simulink model "sampleModel653"  (R2023a)
settings: Solver=VariableStepAuto  StartTime=0.0  StopTime=10.0  RelTol=1e-3
undefined symbols (not defined in the file): DiscIntNeverNeededParam, magnitude, Newton, Raphson
libraries: simulink x238, slpidlib x68
(part 1 of 11)
settings Model: Creator=TSMC  LastModifiedBy=TSMC

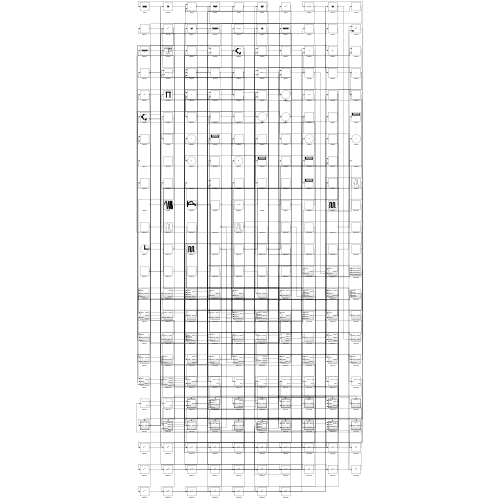
[thumbnail: Simulink's stored preview of the top-level diagram]
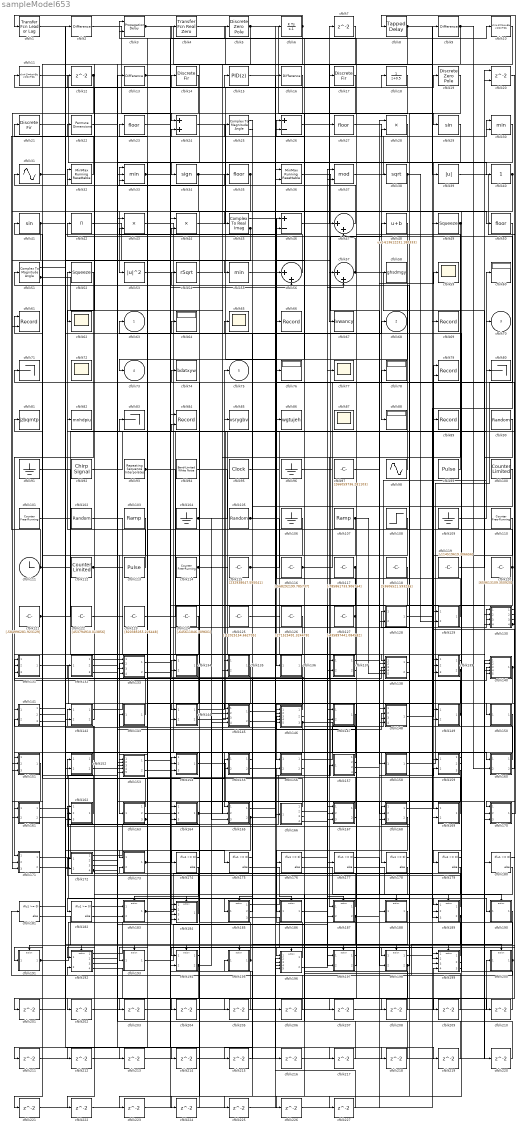
== system sampleModel653 ==
  cfblk1 : simulink/Discrete/Transfer Fcn Lead or Lag  PoleZ=0.95  ZeroZ=0.75  ICPrevOutput=0.0  ICPrevInput=0.0  DoSatur=off
  cfblk10 : DiscreteStateSpace
  cfblk100 : simulink/Sources/Counter Limited  uplimit=[350.000000]  tsamp=-1
  cfblk101 : simulink/Sources/Counter Free-Running  NumBits=[6.000000]  tsamp=-1
  cfblk102 : RandomNumber  Mean=[-2510.054914]  Variance=[85353.178897]  Seed=[22807795.000000]  SampleTime=0.1
  cfblk103 : simulink/Sources/Ramp  slope=[-6750.741057]  start=[19.762170]  InitialOutput=[686609.010483]
  cfblk{91,96,104,106,109} (5 alike) : Ground
  cfblk105 : RandomNumber  Mean=[90146.869558]  Variance=[81141.982069]  Seed=[567805556.000000]  SampleTime=0.1
  cfblk107 : simulink/Sources/Ramp  slope=[382.621128]  start=[12.088717]  InitialOutput=[440961.577354]
  cfblk108 : Step  Time=[7.000000]  Before=[-368987088.994321]  After=[512056900.809752]  SampleTime=0
  cfblk11 : DiscreteStateSpace
  cfblk110 : simulink/Sources/Counter Free-Running  NumBits=[23.000000]  tsamp=-1
  cfblk111 : Clock
  cfblk112 : simulink/Sources/Counter Limited  uplimit=[312.000000]  tsamp=-1
  cfblk113 : DiscretePulseGenerator  PulseType=Time based  Amplitude=[570954732.340234]  Period=[80381016.337612]  PulseWidth=5  PhaseDelay=[1.000000]
  cfblk114 : simulink/Sources/Counter Free-Running  NumBits=[6.000000]  tsamp=-1
  cfblk115 : Constant  Value=[232938647.595041]  SampleTime=1
  cfblk116 : Constant  Value=[-568292199.785737]  SampleTime=1
  cfblk117 : Constant  Value=[-785861733.906764]  SampleTime=1
  cfblk118 : Constant  Value=[53606521.593236]  SampleTime=1
  cfblk119 : Constant  Value=[-114519619.306656]  SampleTime=1
  cfblk{7,12,201..227} (29 alike) : Delay  SampleTime=1
  cfblk120 : Constant  Value=[659613109.350920]  SampleTime=1
  cfblk121 : Constant  Value=[-584996281.923129]  SampleTime=1
  cfblk122 : Constant  Value=[453794910.013856]  SampleTime=1
  cfblk123 : Constant  Value=[820385055.226448]  SampleTime=1
  cfblk124 : Constant  Value=[-645611846.309601]  SampleTime=1
  cfblk125 : Constant  Value=[-12025154.662705]  SampleTime=1
  cfblk126 : Constant  Value=[271525491.324478]  SampleTime=1
  cfblk127 : Constant  Value=[-435897441.084582]  SampleTime=1
  cfblk128 : Subsystem
  cfblk129 : Subsystem
  cfblk{2,9,13,16} (4 alike) : simulink/Discrete/Difference  ICPrevInput=0.0  OutMin=[]  OutMax=[]  OutDataTypeStr=Inherit: Inherit via back propagation  OutDataType=fixdt(1, 16)  OutScaling=2^-10  DoSatur=off
  cfblk130 : Subsystem
  cfblk131 : Subsystem
  cfblk132 : Subsystem
  cfblk133 : Subsystem
  cfblk134 : Subsystem
  cfblk135 : Subsystem
  cfblk136 : Subsystem
  cfblk137 : Subsystem
  cfblk138 : Subsystem
  cfblk139 : Subsystem
  cfblk14 : DiscreteFir  SampleTime=1
  cfblk140 : Subsystem
  cfblk141 : Subsystem
  cfblk142 : Subsystem
  cfblk143 : Subsystem
  cfblk144 : Subsystem
  cfblk145 : Subsystem
  cfblk146 : Subsystem
  cfblk147 : Subsystem
  cfblk148 : Subsystem
  cfblk149 : Subsystem
  cfblk15 : slpidlib/PID Controller  Controller=PID  Form=Parallel  TimeDomain=Discrete-time  UseExternalTs=off  SampleTime=1  IntegratorMethod=Forward Euler  FilterMethod=Forward Euler  ControllerParametersSource=internal  P=1  I=1  UseKiTs=off  D=0  N=100  UseFilter=on  TunerSelectOption=Transfer Function Based (PID Tuner App)  InitialConditionSource=internal  InitialConditionForIntegrator=0  InitialConditionForFilter=0  DifferentiatorICPrevScaledInput=0  ExternalReset=none  TrackingMode=off  Kt=1  LimitOutput=off  SatLimitsSource=internal  UpperSaturationLimit=inf  LowerSaturationLimit=-inf  LinearizeAsGain=off  AntiWindupMode=none  Kb=1  LimitIntegrator=off  UpperIntegratorSaturationLimit=inf  LowerIntegratorSaturationLimit=-inf  POutMin=[]  POutMax=[]  IOutMin=[]  IOutMax=[]  DOutMin=[]  DOutMax=[]  NOutMin=[]  NOutMax=[]  SumOutMin=[]  SumOutMax=[]  SaturationOutMin=[]  SaturationOutMax=[]  PParamMin=[]  PParamMax=[]  IParamMin=[]  IParamMax=[]  DParamMin=[]  DParamMax=[]  NParamMin=[]  NParamMax=[]  KbParamMin=[]  KbParamMax=[]  KtParamMin=[]  KtParamMax=[]  KbOutMin=[]  KbOutMax=[]  KtOutMin=[]  KtOutMax=[]  IntegratorOutMin=[]  IntegratorOutMax=[]  FilterOutMin=[]  FilterOutMax=[]  SumI1OutMin=[]  SumI1OutMax=[]  SumI2OutMin=[]  SumI2OutMax=[]  SumI3OutMin=[]  SumI3OutMax=[]  SumI4OutMin=[]  SumI4OutMax=[]  SumDOutMin=[]  SumDOutMax=[]  DifferentiatorOutMin=[]  DifferentiatorOutMax=[]  FilterDiffOutCoefMin=[]  FilterDiffOutCoefMax=[]  ReciprocalOutMin=[]  ReciprocalOutMax=[]  SumDenOutMin=[]  SumDenOutMax=[]  SumNumOutMin=[]  SumNumOutMax=[]  DivideOutMin=[]  DivideOutMax=[]  UdiffTsProdOutMin=[]  UdiffTsProdOutMax=[]  NTsProdOutMin=[]  NTsProdOutMax=[]  UintegralTsProdOutMin=[]  UintegralTsProdOutMax=[]  UngainTsProdOutMin=[]  UngainTsProdOutMax=[]  ClampingZeroOutDataTypeStr=Inherit: Inherit via back propagation  ClampingZeroOutMin=[]  ClampingZeroOutMax=[]  FilterDenConstantOutDataTypeStr=Inherit: Inherit via back propagation  FilterDenConstantOutMin=[]  FilterDenConstantOutMax=[]  PCopyOutDataTypeStr=Inherit: Inherit via back propagation  PCopyOutMin=[]  PCopyOutMax=[]  NCopyOutDataTypeStr=Inherit: Inherit via back propagation  NCopyOutMin=[]  NCopyOutMax=[]  IntegratorContinuousStateAttributes=''  IntegratorStateMustResolveToSignalObject=off  IntegratorRTWStateStorageClass=Auto  FilterContinuousStateAttributes=''  FilterStateMustResolveToSignalObject=off  FilterRTWStateStorageClass=Auto  ParallelPVariant=InternalParameters  IdealPVariant=Disabled  IVariant=InternalParameters  DVariant=InternalParameters  IntegratorVariant=Discrete  SatVariant=Disabled  AWVariant=Passthrough  PCopyVariant=Disabled  TRVariant=Disabled  FdbkBlocksVariant=Forward  IdealPFdbkVariant=Disabled  SatFdbkVariant=Disabled  DerivativeFilterVariant=ForwardEulerFilter  NVariant=InternalParameters  NCopyVariant=Disabled  FilterICVariant=InternalICsFilter  IntegratorICVariant=InternalICs  ExternalResetVariant=Disabled  TRSumVariant=Passthrough  SumFdbkVariant=Disabled  SumVariant=Sum_PID  TsampFilterVariant=InternalTs  TsampNgainVariant=Passthrough  TsampIntegralVariant=Disabled_SignalSpec  ExternalSaturationOutDataTypeStr=Inherit: Same as second input
      settings: LibrarySourceBlock=simulink/Discrete/Discrete PID Controller
  cfblk150 : Subsystem
  cfblk151 : Subsystem
  cfblk152 : Subsystem
  cfblk153 : Subsystem
  cfblk154 : Subsystem
  cfblk155 : Subsystem
  cfblk156 : Subsystem
  cfblk157 : Subsystem
  cfblk158 : Subsystem
  cfblk159 : Subsystem
  cfblk160 : Subsystem
  cfblk161 : Subsystem
  cfblk162 : Subsystem
  cfblk163 : Subsystem
  cfblk164 : Subsystem
  cfblk165 : Subsystem
  cfblk166 : Subsystem
  cfblk167 : Subsystem
  cfblk168 : Subsystem
  cfblk169 : Subsystem
  cfblk17 : DiscreteFir  SampleTime=1
  cfblk170 : Subsystem
  cfblk171 : Subsystem
  cfblk172 : Subsystem
  cfblk173 : Subsystem
  cfblk{174..182} (9 alike) : If  IfExpression=u1 >= 0  SampleTime=1
  cfblk18 : DiscreteTransferFcn  SampleTime=1
  cfblk183 : Subsystem  TreatAsAtomicUnit=on
  cfblk184 : Subsystem  TreatAsAtomicUnit=on
  cfblk185 : Subsystem  TreatAsAtomicUnit=on
  cfblk186 : Subsystem  TreatAsAtomicUnit=on
  cfblk187 : Subsystem  TreatAsAtomicUnit=on
  cfblk188 : Subsystem  TreatAsAtomicUnit=on
  cfblk189 : Subsystem  TreatAsAtomicUnit=on
  cfblk19 : DiscreteZeroPole  Poles=[0 0.5]  Gain=1
  cfblk190 : Subsystem  TreatAsAtomicUnit=on
  cfblk191 : Subsystem  TreatAsAtomicUnit=on
  cfblk192 : Subsystem  TreatAsAtomicUnit=on
  cfblk193 : Subsystem  TreatAsAtomicUnit=on
  cfblk194 : Subsystem  TreatAsAtomicUnit=on
  cfblk195 : Subsystem  TreatAsAtomicUnit=on
  cfblk196 : Subsystem  TreatAsAtomicUnit=on
  cfblk197 : Subsystem  TreatAsAtomicUnit=on
  cfblk198 : Subsystem  TreatAsAtomicUnit=on
  cfblk199 : Subsystem  TreatAsAtomicUnit=on
  cfblk20 : Delay  ShowEnablePort=on  SampleTime=1
      settings: InputPortMap=u0,e6
  cfblk200 : Subsystem  TreatAsAtomicUnit=on
  cfblk21 : DiscreteFir  SampleTime=1
  cfblk22 : PermuteDimensions
  cfblk{23,27,35,50} (4 alike) : Rounding
  cfblk24 : Sum
  cfblk25 : ComplexToMagnitudeAngle
  cfblk26 : Sum  Inputs=+-
  cfblk28 : Product
  cfblk29 : Trigonometry
  cfblk3 : PropagationDelay  SampleTime=1
  cfblk30 : MinMax  Inputs=2
  cfblk31 : Sin  TimeSource=Use external signal  SampleTime=0
  cfblk32 : simulink/Math Operations/MinMax Running Resettable  Function=min  vinit=0.0
  cfblk33 : MinMax  Inputs=3
  cfblk34 : Signum
  cfblk36 : simulink/Math Operations/MinMax Running Resettable  Function=min  vinit=0.0
  cfblk37 : Math  Operator=mod
  cfblk38 : Sqrt
  cfblk39 : Abs  SaturateOnIntegerOverflow=off
  cfblk4 : simulink/Discrete/Transfer Fcn Real Zero  ZeroZ=0.75  ICPrevInput=0.0  DoSatur=off
  cfblk40 : simulink/Math Operations/Slider Gain  gain=1  low=0  high=2
  cfblk41 : Trigonometry
  cfblk42 : Product  Inputs=*
  cfblk43 : Product  Inputs=**
  cfblk44 : Product  Inputs=**
  cfblk45 : ComplexToRealImag
  cfblk46 : Sum  Inputs=+-
  cfblk47 : Sum  Inputs=|++
  cfblk48 : Bias  Bias=[-613612231.180333]  SaturateOnIntegerOverflow=off
  cfblk49 : Squeeze
  cfblk5 : DiscreteZeroPole  Poles=[0 0.5]  Gain=1
  cfblk51 : ComplexToMagnitudeAngle
  cfblk52 : Squeeze
  cfblk53 : Math  Operator=magnitude^2
  cfblk54 : Sqrt  Operator=rSqrt  AlgorithmType=Newton-Raphson
  cfblk55 : MinMax
  cfblk56 : Sum  Inputs=|++
  cfblk57 : Sum  Inputs=|++
  cfblk58 : ToWorkspace  VariableName=ghsdmgy  SaveFormat=Timeseries  SampleTime=-1
  cfblk{59,62,65,72,77,87} (6 alike) : Scope
      cfblk72 settings: Floating=on
      cfblk87 settings: Floating=on
  cfblk6 : DiscreteIntegrator  ICPrevOutput=DiscIntNeverNeededParam  ICPrevScaledInput=DiscIntNeverNeededParam
  cfblk{60,64,76,78,88} (5 alike) : Display
  cfblk61 : Record  FileSettingsInternal="{\"entries\":[{\"content\":{\"excelSettings\":{\"content\":{},\"type\":\"Streamout.ExcelSettings\"}},\"type\":\"Streamout.FileSettingStorage\",\"uuid\":\"\"}],\"packageUris\":[\"http:\\/\\/schema.mathworks.com\\/mf0\\/streamout_blocks\\/R2020a\"],\"version\":\"1.0\"}"  Layout=[1 1]  SignalsInternal="{\"entries\":[{\"content\":{\"signals\":[{\"content\":{\"blockPath\":[],\"dimensions\":[1],\"domain\":\"\",\"lineColor\":\"#a2142f\",\"plots\":[1],\"port\":1,\"signalID\":35743,\"signalName\":\"XY Graph:1\"},\"type\":\"RecordBlkView.Signal\",\"uuid\":\"\"},{\"content\":{\"blockPath\":[],\"dimensions\":[1],\"domain\":\"\",\"lineColor\":\"#139fff\",\"plots\":[1],\"port\":2,\"signalID\":35746,\"signalName\":\"XY Graph:2\"},\"type\":\"RecordBlkView.Signal\",\"uuid\":\"\"}]},\"type\":\"RecordBlkView.InputSignals\",\"uuid\":\"\"}],\"packageUris\":[\"http:\\/\\/schema.mathworks.com\\/mf0\\/streamout_blocks\\/R2020a\"],\"version\":\"1.0\"}"  VisualizationBindings="{\"xyplotplugin\":{\"info\":[{\"series\":[{\"bindingParametersList\":[{\"parameter\":\"X-Axis\",\"signalID\":35743,\"signalName\":\"XY Graph:1\"},{\"parameter\":\"Y-Axis\",\"signalID\":35746,\"signalName\":\"XY Graph:2\"}],\"seriesID\":38443}],\"subplotID\":1}]}}"  CompatibilityTag=XY
  cfblk66 : Record  FileSettingsInternal="{\"entries\":[{\"content\":{\"excelSettings\":{\"content\":{},\"type\":\"Streamout.ExcelSettings\"}},\"type\":\"Streamout.FileSettingStorage\",\"uuid\":\"\"}],\"packageUris\":[\"http:\\/\\/schema.mathworks.com\\/mf0\\/streamout_blocks\\/R2020a\"],\"version\":\"1.0\"}"  SignalsInternal="{\"entries\":[{\"content\":{},\"type\":\"RecordBlkView.InputSignals\",\"uuid\":\"\"}],\"packageUris\":[\"http:\\/\\/schema.mathworks.com\\/mf0\\/streamout_blocks\\/R2020a\"],\"version\":\"1.0\"}"  VisualizationBindings="{\"sparklinesplugin\":{\"info\":[{\"bindingParametersList\":[],\"subplotID\":1}]}}"
  cfblk67 : ToWorkspace  VariableName=lvwancy  SaveFormat=Timeseries  SampleTime=-1
  cfblk69 : Record  FileSettingsInternal="{\"entries\":[{\"content\":{\"excelSettings\":{\"content\":{},\"type\":\"Streamout.ExcelSettings\"}},\"type\":\"Streamout.FileSettingStorage\",\"uuid\":\"\"}],\"packageUris\":[\"http:\\/\\/schema.mathworks.com\\/mf0\\/streamout_blocks\\/R2020a\"],\"version\":\"1.0\"}"  SignalsInternal="{\"entries\":[{\"content\":{},\"type\":\"RecordBlkView.InputSignals\",\"uuid\":\"\"}],\"packageUris\":[\"http:\\/\\/schema.mathworks.com\\/mf0\\/streamout_blocks\\/R2020a\"],\"version\":\"1.0\"}"  VisualizationBindings="{\"sparklinesplugin\":{\"info\":[{\"bindingParametersList\":[],\"subplotID\":1}]}}"
  cfblk71 : Terminator
  cfblk74 : ToWorkspace  VariableName=bdatxyw  SaveFormat=Timeseries  SampleTime=-1
  cfblk79 : Record  FileSettingsInternal="{\"entries\":[{\"content\":{\"excelSettings\":{\"content\":{},\"type\":\"Streamout.ExcelSettings\"}},\"type\":\"Streamout.FileSettingStorage\",\"uuid\":\"\"}],\"packageUris\":[\"http:\\/\\/schema.mathworks.com\\/mf0\\/streamout_blocks\\/R2020a\"],\"version\":\"1.0\"}"  Layout=[1 1]  SignalsInternal="{\"entries\":[{\"content\":{\"signals\":[{\"content\":{\"blockPath\":[],\"dimensions\":[1],\"domain\":\"\",\"lineColor\":\"#a2142f\",\"plots\":[1],\"port\":1,\"signalID\":35751,\"signalName\":\"XY Graph:1\"},\"type\":\"RecordBlkView.Signal\",\"uuid\":\"\"},{\"content\":{\"blockPath\":[],\"dimensions\":[1],\"domain\":\"\",\"lineColor\":\"#139fff\",\"plots\":[1],\"port\":2,\"signalID\":35754,\"signalName\":\"XY Graph:2\"},\"type\":\"RecordBlkView.Signal\",\"uuid\":\"\"}]},\"type\":\"RecordBlkView.InputSignals\",\"uuid\":\"\"}],\"packageUris\":[\"http:\\/\\/schema.mathworks.com\\/mf0\\/streamout_blocks\\/R2020a\"],\"version\":\"1.0\"}"  VisualizationBindings="{\"xyplotplugin\":{\"info\":[{\"series\":[{\"bindingParametersList\":[{\"parameter\":\"X-Axis\",\"signalID\":35751,\"signalName\":\"XY Graph:1\"},{\"parameter\":\"Y-Axis\",\"signalID\":35754,\"signalName\":\"XY Graph:2\"}],\"seriesID\":62220}],\"subplotID\":1}]}}"  CompatibilityTag=XY
  cfblk8 : simulink/Discrete/Tapped Delay  vinit=0.0  samptime=-1  NumDelays=1  DelayOrder=Oldest  includeCurrent=off
  cfblk80 : Terminator
  cfblk81 : ToWorkspace  VariableName=jzbqmtp  SaveFormat=Timeseries  SampleTime=-1
  cfblk82 : ToWorkspace  VariableName=mnhdpiu  SaveFormat=Timeseries  SampleTime=-1
  cfblk83 : Terminator
  cfblk84 : Record  FileSettingsInternal="{\"entries\":[{\"content\":{\"excelSettings\":{\"content\":{},\"type\":\"Streamout.ExcelSettings\"}},\"type\":\"Streamout.FileSettingStorage\",\"uuid\":\"\"}],\"packageUris\":[\"http:\\/\\/schema.mathworks.com\\/mf0\\/streamout_blocks\\/R2020a\"],\"version\":\"1.0\"}"  Layout=[1 1]  SignalsInternal="{\"entries\":[{\"content\":{\"signals\":[{\"content\":{\"blockPath\":[],\"dimensions\":[1],\"domain\":\"\",\"lineColor\":\"#a2142f\",\"plots\":[1],\"port\":1,\"signalID\":35759,\"signalName\":\"XY Graph:1\"},\"type\":\"RecordBlkView.Signal\",\"uuid\":\"\"},{\"content\":{\"blockPath\":[],\"dimensions\":[1],\"domain\":\"\",\"lineColor\":\"#139fff\",\"plots\":[1],\"port\":2,\"signalID\":35762,\"signalName\":\"XY Graph:2\"},\"type\":\"RecordBlkView.Signal\",\"uuid\":\"\"}]},\"type\":\"RecordBlkView.InputSignals\",\"uuid\":\"\"}],\"packageUris\":[\"http:\\/\\/schema.mathworks.com\\/mf0\\/streamout_blocks\\/R2020a\"],\"version\":\"1.0\"}"  VisualizationBindings="{\"xyplotplugin\":{\"info\":[{\"series\":[{\"bindingParametersList\":[{\"parameter\":\"X-Axis\",\"signalID\":35759,\"signalName\":\"XY Graph:1\"},{\"parameter\":\"Y-Axis\",\"signalID\":35762,\"signalName\":\"XY Graph:2\"}],\"seriesID\":44318}],\"subplotID\":1}]}}"  CompatibilityTag=XY
  cfblk85 : ToWorkspace  VariableName=vsrygbv  SaveFormat=Timeseries  SampleTime=-1
  cfblk86 : ToWorkspace  VariableName=wgtujeh  SaveFormat=Timeseries  SampleTime=-1
  cfblk89 : Record  FileSettingsInternal="{\"entries\":[{\"content\":{\"excelSettings\":{\"content\":{},\"type\":\"Streamout.ExcelSettings\"}},\"type\":\"Streamout.FileSettingStorage\",\"uuid\":\"\"}],\"packageUris\":[\"http:\\/\\/schema.mathworks.com\\/mf0\\/streamout_blocks\\/R2020a\"],\"version\":\"1.0\"}"  SignalsInternal="{\"entries\":[{\"content\":{},\"type\":\"RecordBlkView.InputSignals\",\"uuid\":\"\"}],\"packageUris\":[\"http:\\/\\/schema.mathworks.com\\/mf0\\/streamout_blocks\\/R2020a\"],\"version\":\"1.0\"}"  VisualizationBindings="{\"sparklinesplugin\":{\"info\":[{\"bindingParametersList\":[],\"subplotID\":1}]}}"
  cfblk90 : RandomNumber  Mean=[81983.003222]  Variance=[14220.056045]  Seed=[398225088.000000]  SampleTime=0.1
  cfblk92 : simulink/Sources/Chirp Signal  f1=[-164452371.357946]  T=[-247135005.835432]  f2=[-278737308.417213]
  cfblk93 : simulink/Sources/Repeating Sequence Interpolated  OutValues=[-576342041.016997, 372535724.917428, 895075316.780555, 485237690.974424, -398965901.988009]  TimeValues=[0 0.1 0.5 0.6 1].'  LookUpMeth=Use Input Above  tsamp=0.01  OutMin=[]  OutMax=[]  OutDataTypeStr=double  OutputDataTypeScalingMode=double  OutDataType=fixdt(0,8)  OutScaling=2^-10
  cfblk94 : simulink/Sources/Band-Limited White Noise  Cov=[3370681036.098789]  Ts=0.1  seed=[9057757928.000000]
  cfblk95 : DigitalClock
  cfblk97 : Constant  Value=[266059736.281103]  SampleTime=1
  cfblk98 : Sin  Amplitude=[-992289981.566664]  Bias=[-48582616.764596]  SampleTime=0
  cfblk99 : DiscretePulseGenerator  PulseType=Time based  Amplitude=[883932493.982102]  Period=[82177714.004234]  PulseWidth=5  PhaseDelay=[9.000000]
  cfblk63 : Outport
  cfblk68 : Outport  Port=2
  cfblk70 : Outport  Port=3
  cfblk73 : Outport  Port=4
  cfblk75 : Outport  Port=5
  wires:
  cfblk192/1(cfblk2) -> cfblk154/1(cfblk1)
  cfblk98/1 -> cfblk51/1
  cfblk2/1 -> cfblk24/1
  cfblk156/1(cfblk2) -> cfblk60/1
  cfblk44/1 -> cfblk19/1
  cfblk136/1(cfblk2) -> cfblk156/1(cfblk1)
  cfblk111/1 -> cfblk24/2, cfblk153/5(cfblk15)
  cfblk158/1(cfblk2) -> cfblk42/1
  cfblk45/1 -> cfblk136/1(cfblk1)
  cfblk127/1 -> cfblk46/1, cfblk145/1(cfblk1)
  cfblk51/1 -> cfblk2/1
  cfblk169/1(cfblk2) -> cfblk71/1
  cfblk99/1 -> cfblk32/1
  cfblk39/1 -> cfblk150/1(cfblk1)
  cfblk109/1 -> cfblk70/1
  cfblk49/1 -> cfblk187/1(cfblk1), cfblk145/3(cfblk14)
  cfblk118/1 -> cfblk154/2(cfblk12)
  cfblk147/1(cfblk2) -> cfblk174/1
  cfblk196/1(cfblk2) -> cfblk156/2(cfblk15)
  cfblk107/1 -> cfblk163/1(cfblk1), cfblk138/5(cfblk16)
  cfblk126/1 -> cfblk171/1(cfblk1)
  cfblk26/1 -> cfblk7/1
  cfblk27/1 -> cfblk88/1
  cfblk43/1 -> cfblk197/1(cfblk1)
  cfblk144/1(cfblk2) -> cfblk75/1
  cfblk129/1(cfblk2) -> cfblk26/1
  cfblk23/1 -> cfblk164/1(cfblk1)
  cfblk170/1(cfblk2) -> cfblk8/1
  cfblk11/1 -> cfblk169/1(cfblk1)
  cfblk148/1(cfblk2) -> cfblk79/1
  cfblk156/2(cfblk16) -> cfblk32/2
  cfblk197/2(cfblk10) -> cfblk15/1
  cfblk172/1(cfblk2) -> cfblk48/1
  cfblk135/1(cfblk2) -> cfblk164/2(cfblk7)
  cfblk116/1 -> cfblk20/1, cfblk89/1
  cfblk150/1(cfblk2) -> cfblk165/1(cfblk1)
  cfblk53/1 -> cfblk178/1
  cfblk168/1(cfblk2) -> cfblk49/1
  cfblk119/1 -> cfblk20/2
  cfblk160/1(cfblk2) -> cfblk54/1
  cfblk41/1 -> cfblk160/1(cfblk1), cfblk171/3(cfblk9)
  cfblk139/1(cfblk2) -> cfblk154/3(cfblk13)
  cfblk47/1 -> cfblk22/1
  cfblk34/1 -> cfblk86/1, cfblk144/2(cfblk7)
  cfblk113/1 -> cfblk52/1
  cfblk91/1 -> cfblk166/1(cfblk1)
  cfblk31/1 -> cfblk14/1, cfblk148/4(cfblk8)
  cfblk162/1(cfblk2) -> cfblk61/1
  cfblk32/1 -> cfblk21/1
  cfblk7/1 -> cfblk34/1
  cfblk105/1 -> cfblk65/1, cfblk140/2(cfblk7)
  cfblk183/1(cfblk2) -> cfblk69/1, cfblk140/3(cfblk8)
  cfblk138/1(cfblk2) -> cfblk182/1
  cfblk184/1(cfblk2) -> cfblk142/1(cfblk1)
  cfblk3/1 -> cfblk39/1, cfblk196/1(cfblk1)
  cfblk51/2 -> cfblk165/2(cfblk8), cfblk46/2
  cfblk189/1(cfblk2) -> cfblk168/1(cfblk1)
  cfblk4/1 -> cfblk67/1
  cfblk30/1 -> cfblk76/1
  cfblk6/1 -> cfblk1/1, cfblk135/2(cfblk10)
  cfblk138/2(cfblk17) -> cfblk198/1(cfblk1)
  cfblk96/1 -> cfblk9/1
  cfblk106/1 -> cfblk191/1(cfblk1)
  cfblk193/1(cfblk2) -> cfblk167/1(cfblk1)
  cfblk5/1 -> cfblk29/1, cfblk33/2
  cfblk196/2(cfblk17) -> cfblk77/1
  cfblk133/1(cfblk2) -> cfblk164/3(cfblk8)
  cfblk124/1 -> cfblk193/1(cfblk1)
  cfblk190/1(cfblk2) -> cfblk181/1
  cfblk165/1(cfblk2) -> cfblk198/2(cfblk16)
  cfblk167/1(cfblk2) -> cfblk143/1(cfblk1)
  cfblk93/1 -> cfblk138/1(cfblk1), cfblk130/4(cfblk13)
  cfblk134/1(cfblk2) -> cfblk173/1(cfblk1)
  cfblk168/2(cfblk12) -> cfblk186/1(cfblk1)
  cfblk29/1 -> cfblk153/1(cfblk1)
  cfblk35/1 -> cfblk144/1(cfblk1), cfblk33/3
  cfblk38/1 -> cfblk53/1, cfblk129/2(cfblk13)
  cfblk142/1(cfblk2) -> cfblk149/1(cfblk1)
  cfblk46/1 -> cfblk17/1
  cfblk200/1(cfblk2) -> cfblk128/1(cfblk1), cfblk192/2(cfblk14)
  cfblk40/1 -> cfblk61/2, cfblk209/1
  cfblk130/3(cfblk15) -> cfblk194/1(cfblk1)
  cfblk52/1 -> cfblk141/1(cfblk1)
  cfblk92/1 -> cfblk44/1
  cfblk131/1(cfblk2) -> cfblk146/1(cfblk1)
  cfblk145/1(cfblk2) -> cfblk78/1
  cfblk139/2(cfblk16) -> cfblk64/1, cfblk207/1
  cfblk33/1 -> cfblk28/2, cfblk47/1, cfblk218/1
  cfblk185/1(cfblk2) -> cfblk190/1(cfblk1)
  cfblk140/1(cfblk2) -> cfblk179/1, cfblk213/1
  cfblk112/1 -> cfblk12/1, cfblk187/2(cfblk6)
  cfblk37/1 -> cfblk30/1
  cfblk9/1 -> cfblk151/1(cfblk1), cfblk160/2(cfblk8)
  cfblk137/1(cfblk2) -> cfblk59/1
  cfblk157/1(cfblk2) -> cfblk63/1
  cfblk146/1(cfblk2) -> cfblk82/1
  cfblk104/1 -> cfblk16/1, cfblk165/3(cfblk9)
  cfblk154/1(cfblk2) -> cfblk197/2(cfblk9)
  cfblk120/1 -> cfblk23/1, cfblk147/2(cfblk14)
  cfblk45/2 -> cfblk151/2(cfblk10), cfblk43/2
  cfblk189/2(cfblk10) -> cfblk83/1, cfblk131/3(cfblk15), cfblk227/1
  cfblk28/1 -> cfblk153/2(cfblk12)
  cfblk25/1 -> cfblk45/1
  cfblk123/1 -> cfblk36/1
  cfblk187/1(cfblk2) -> cfblk141/2(cfblk5)
  cfblk195/1(cfblk2) -> cfblk184/2(cfblk13), cfblk162/2(cfblk12)
  cfblk165/2(cfblk10) -> cfblk36/2, cfblk172/2(cfblk6)
  cfblk192/2(cfblk15) -> cfblk44/2
  cfblk173/1(cfblk2) -> cfblk85/1, cfblk33/1
  cfblk153/1(cfblk2) -> cfblk130/1(cfblk1)
  cfblk14/1 -> cfblk161/1(cfblk1)
  cfblk48/1 -> cfblk73/1
  cfblk199/1(cfblk2) -> cfblk66/1
  cfblk145/2(cfblk16) -> cfblk30/2
  cfblk17/1 -> cfblk183/2(cfblk8)
  cfblk108/1 -> cfblk146/2(cfblk9)
  cfblk117/1 -> cfblk167/2(cfblk15), cfblk194/2(cfblk12)
  cfblk171/1(cfblk2) -> cfblk84/1
  cfblk161/1(cfblk2) -> cfblk189/1(cfblk1)
  cfblk146/2(cfblk13) -> cfblk134/1(cfblk1)
  cfblk166/1(cfblk2) -> cfblk152/1(cfblk1)
  cfblk141/1(cfblk2) -> cfblk68/1
  cfblk186/1(cfblk2) -> cfblk37/1
  cfblk94/1 -> cfblk169/2(cfblk7)
  cfblk101/1 -> cfblk26/2
  cfblk12/1 -> cfblk161/2(cfblk15), cfblk151/3(cfblk11)
  cfblk149/1(cfblk2) -> cfblk133/2(cfblk7), cfblk135/1(cfblk1)
  cfblk185/2(cfblk13) -> cfblk134/2(cfblk9)
  cfblk164/1(cfblk2) -> cfblk168/2(cfblk10), cfblk140/5(cfblk10)
  cfblk36/1 -> cfblk128/2(cfblk17)
  cfblk152/1(cfblk2) -> cfblk81/1
  cfblk133/2(cfblk10) -> cfblk175/1
  cfblk171/2(cfblk10) -> cfblk43/1
  cfblk18/1 -> cfblk56/1
  cfblk191/1(cfblk2) -> cfblk5/1, cfblk18/1, cfblk146/4(cfblk11)
  cfblk97/1 -> cfblk158/1(cfblk1)
  cfblk24/1 -> cfblk50/1
  cfblk192/3(cfblk16) -> cfblk25/1
  cfblk121/1 -> cfblk37/2, cfblk80/1
  cfblk157/2(cfblk13) -> cfblk146/3(cfblk10)
  cfblk130/4(cfblk16) -> cfblk74/1, cfblk84/2
  cfblk110/1 -> cfblk189/2(cfblk8)
  cfblk55/1 -> cfblk189/3(cfblk9)
  cfblk172/2(cfblk7) -> cfblk13/1
  cfblk185/3(cfblk14) -> cfblk199/2(cfblk13)
  cfblk57/1 -> cfblk180/1, cfblk47/2
  cfblk142/2(cfblk16) -> cfblk31/1
  cfblk1/1 -> cfblk57/1
  cfblk115/1 -> cfblk57/2, cfblk58/1
  cfblk137/2(cfblk14) -> cfblk4/1
  cfblk20/1 -> cfblk170/1(cfblk1)
  cfblk103/1 -> cfblk153/4(cfblk14)
  cfblk160/2(cfblk9) -> cfblk129/1(cfblk1)
  cfblk166/2(cfblk8) -> cfblk139/1(cfblk1)
  cfblk56/1 -> cfblk3/1
  cfblk157/3(cfblk14) -> cfblk79/2
  cfblk187/2(cfblk7) -> cfblk159/2(cfblk6), cfblk226/1
  cfblk13/1 -> cfblk10/1, cfblk140/4(cfblk9)
  cfblk128/1(cfblk2) -> cfblk139/2(cfblk14)
  cfblk102/1 -> cfblk177/1
  cfblk42/1 -> cfblk55/1
  cfblk50/1 -> cfblk139/3(cfblk15)
  cfblk141/2(cfblk6) -> cfblk137/1(cfblk1)
  cfblk54/1 -> cfblk170/2(cfblk13)
  cfblk122/1 -> cfblk148/1(cfblk1)
  cfblk90/1 -> cfblk130/2(cfblk11)
  cfblk16/1 -> cfblk152/2(cfblk13)
  cfblk146/3(cfblk14) -> cfblk220/1, cfblk221/1
  cfblk152/2(cfblk14) -> cfblk35/1
  cfblk143/1(cfblk2) -> cfblk132/1(cfblk1)
  cfblk166/3(cfblk9) -> cfblk3/2
  cfblk172/3(cfblk8) -> cfblk148/2(cfblk6)
  cfblk100/1 -> cfblk185/1(cfblk1)
  cfblk198/1(cfblk2) -> cfblk159/1(cfblk1)
  cfblk125/1 -> cfblk147/1(cfblk1)
  cfblk198/2(cfblk17) -> cfblk162/1(cfblk1), cfblk225/1
  cfblk8/1 -> cfblk40/1, cfblk162/3(cfblk13)
  cfblk151/1(cfblk2) -> cfblk171/2(cfblk8)
  cfblk95/1 -> cfblk38/1
  cfblk161/2(cfblk16) -> cfblk155/1(cfblk1)
  cfblk159/2(cfblk7) -> cfblk167/3(cfblk16)
  cfblk199/2(cfblk16) -> cfblk155/2(cfblk9)
  cfblk172/4(cfblk9) -> cfblk148/3(cfblk7), cfblk192/1(cfblk1), cfblk222/1
  cfblk132/1(cfblk2) -> cfblk170/3(cfblk14)
  cfblk157/4(cfblk15) -> cfblk131/1(cfblk1)
  cfblk166/4(cfblk10) -> cfblk130/3(cfblk12)
  cfblk144/2(cfblk8) -> cfblk6/1
  cfblk10/1 -> cfblk62/1
  cfblk155/2(cfblk10) -> cfblk157/1(cfblk1)
  cfblk163/1(cfblk2) -> cfblk41/1
  cfblk194/2(cfblk13) -> cfblk145/2(cfblk13), cfblk212/1
  cfblk167/2(cfblk17) -> cfblk11/1
  cfblk199/3(cfblk17) -> cfblk172/1(cfblk1)
  cfblk163/2(cfblk8) -> cfblk56/2
  cfblk114/1 -> cfblk137/2(cfblk13), cfblk145/4(cfblk15)
  cfblk132/3(cfblk14) -> cfblk27/1
  cfblk163/3(cfblk9) -> cfblk133/4(cfblk9), cfblk131/2(cfblk14)
  cfblk141/3(cfblk7) -> cfblk138/3(cfblk14)
  cfblk174/1 -> cfblk183/Action
  cfblk174/2 -> cfblk184/Action
  cfblk175/1 -> cfblk185/Action
  cfblk175/2 -> cfblk186/Action
  cfblk176/1 -> cfblk187/Action
  cfblk176/2 -> cfblk188/Action
  cfblk177/1 -> cfblk189/Action
  cfblk177/2 -> cfblk190/Action
  cfblk178/1 -> cfblk191/Action
  cfblk178/2 -> cfblk192/Action
  cfblk179/1 -> cfblk193/Action
  cfblk179/2 -> cfblk194/Action
  cfblk180/1 -> cfblk195/Action
  cfblk180/2 -> cfblk196/Action
  cfblk181/1 -> cfblk197/Action
  cfblk181/2 -> cfblk198/Action
  cfblk182/1 -> cfblk199/Action
  cfblk182/2 -> cfblk200/Action
  cfblk155/1(cfblk2) -> cfblk201/1
  cfblk201/1 -> cfblk142/2(cfblk15)
  cfblk130/1(cfblk2) -> cfblk202/1
  cfblk202/1 -> cfblk199/1(cfblk1)
  cfblk130/2(cfblk14) -> cfblk203/1
  cfblk203/1 -> cfblk200/1(cfblk1)
  cfblk197/1(cfblk2) -> cfblk204/1
  cfblk204/1 -> cfblk188/1(cfblk1)
  cfblk188/1(cfblk2) -> cfblk205/1
  cfblk205/1 -> cfblk184/3(cfblk14)
  cfblk15/1 -> cfblk206/1
  cfblk206/1 -> cfblk153/3(cfblk13)
  cfblk207/1 -> cfblk199/4(cfblk15)
  cfblk19/1 -> cfblk208/1
  cfblk208/1 -> cfblk183/1(cfblk1)
  cfblk209/1 -> cfblk146/5(cfblk12)
  cfblk132/2(cfblk13) -> cfblk210/1
  cfblk210/1 -> cfblk173/2(cfblk7)
  cfblk194/1(cfblk2) -> cfblk211/1
  cfblk211/1 -> cfblk140/1(cfblk1)
  cfblk212/1 -> cfblk168/3(cfblk11)
  cfblk213/1 -> cfblk196/3(cfblk14)
  cfblk21/1 -> cfblk214/1
  cfblk214/1 -> cfblk28/1
  cfblk25/2 -> cfblk215/1
  cfblk215/1 -> cfblk195/1(cfblk1)
  cfblk192/4(cfblk17) -> cfblk216/1
  cfblk216/1 -> cfblk138/2(cfblk13)
  cfblk153/2(cfblk16) -> cfblk217/1
  cfblk217/1 -> cfblk176/1
  cfblk218/1 -> cfblk196/2(cfblk13)
  cfblk22/1 -> cfblk219/1
  cfblk219/1 -> cfblk133/1(cfblk1)
  cfblk220/1 -> cfblk133/3(cfblk8)
  cfblk221/1 -> cfblk138/4(cfblk15)
  cfblk222/1 -> cfblk199/3(cfblk14)
  cfblk159/1(cfblk2) -> cfblk223/1
  cfblk223/1 -> cfblk184/1(cfblk1)
  cfblk159/3(cfblk8) -> cfblk224/1
  cfblk224/1 -> cfblk184/4(cfblk15)
  cfblk225/1 -> cfblk196/5(cfblk16)
  cfblk226/1 -> cfblk149/2(cfblk15)
  cfblk227/1 -> cfblk196/4(cfblk15)

== system sampleModel653/cfblk128 ==
  cfblk1 : Inport
  cfblk17 : Inport  Port=2
  cfblk10 : Math  Operator=mod
  cfblk11 : Constant  Value=[-332037826.006319]  SampleTime=1
  cfblk12 : Subsystem
  cfblk13 : Subsystem
  cfblk14 : Subsystem
  cfblk15 : Subsystem
  cfblk16 : Subsystem
  cfblk18 : Delay  SampleTime=1
  cfblk19 : Delay  SampleTime=1
  cfblk3 : slpidlib/PID Controller  Controller=PID  Form=Parallel  TimeDomain=Discrete-time  UseExternalTs=off  SampleTime=1  IntegratorMethod=Forward Euler  FilterMethod=Forward Euler  ControllerParametersSource=internal  P=1  I=1  UseKiTs=off  D=0  N=100  UseFilter=on  TunerSelectOption=Transfer Function Based (PID Tuner App)  InitialConditionSource=internal  InitialConditionForIntegrator=0  InitialConditionForFilter=0  DifferentiatorICPrevScaledInput=0  ExternalReset=none  TrackingMode=off  Kt=1  LimitOutput=off  SatLimitsSource=internal  UpperSaturationLimit=inf  LowerSaturationLimit=-inf  LinearizeAsGain=off  AntiWindupMode=none  Kb=1  LimitIntegrator=off  UpperIntegratorSaturationLimit=inf  LowerIntegratorSaturationLimit=-inf  POutMin=[]  POutMax=[]  IOutMin=[]  IOutMax=[]  DOutMin=[]  DOutMax=[]  NOutMin=[]  NOutMax=[]  SumOutMin=[]  SumOutMax=[]  SaturationOutMin=[]  SaturationOutMax=[]  PParamMin=[]  PParamMax=[]  IParamMin=[]  IParamMax=[]  DParamMin=[]  DParamMax=[]  NParamMin=[]  NParamMax=[]  KbParamMin=[]  KbParamMax=[]  KtParamMin=[]  KtParamMax=[]  KbOutMin=[]  KbOutMax=[]  KtOutMin=[]  KtOutMax=[]  IntegratorOutMin=[]  IntegratorOutMax=[]  FilterOutMin=[]  FilterOutMax=[]  SumI1OutMin=[]  SumI1OutMax=[]  SumI2OutMin=[]  SumI2OutMax=[]  SumI3OutMin=[]  SumI3OutMax=[]  SumI4OutMin=[]  SumI4OutMax=[]  SumDOutMin=[]  SumDOutMax=[]  DifferentiatorOutMin=[]  DifferentiatorOutMax=[]  FilterDiffOutCoefMin=[]  FilterDiffOutCoefMax=[]  ReciprocalOutMin=[]  ReciprocalOutMax=[]  SumDenOutMin=[]  SumDenOutMax=[]  SumNumOutMin=[]  SumNumOutMax=[]  DivideOutMin=[]  DivideOutMax=[]  UdiffTsProdOutMin=[]  UdiffTsProdOutMax=[]  NTsProdOutMin=[]  NTsProdOutMax=[]  UintegralTsProdOutMin=[]  UintegralTsProdOutMax=[]  UngainTsProdOutMin=[]  UngainTsProdOutMax=[]  ClampingZeroOutDataTypeStr=Inherit: Inherit via back propagation  ClampingZeroOutMin=[]  ClampingZeroOutMax=[]  FilterDenConstantOutDataTypeStr=Inherit: Inherit via back propagation  FilterDenConstantOutMin=[]  FilterDenConstantOutMax=[]  PCopyOutDataTypeStr=Inherit: Inherit via back propagation  PCopyOutMin=[]  PCopyOutMax=[]  NCopyOutDataTypeStr=Inherit: Inherit via back propagation  NCopyOutMin=[]  NCopyOutMax=[]  IntegratorContinuousStateAttributes=''  IntegratorStateMustResolveToSignalObject=off  IntegratorRTWStateStorageClass=Auto  FilterContinuousStateAttributes=''  FilterStateMustResolveToSignalObject=off  FilterRTWStateStorageClass=Auto  ParallelPVariant=InternalParameters  IdealPVariant=Disabled  IVariant=InternalParameters  DVariant=InternalParameters  IntegratorVariant=Discrete  SatVariant=Disabled  AWVariant=Passthrough  PCopyVariant=Disabled  TRVariant=Disabled  FdbkBlocksVariant=Forward  IdealPFdbkVariant=Disabled  SatFdbkVariant=Disabled  DerivativeFilterVariant=ForwardEulerFilter  NVariant=InternalParameters  NCopyVariant=Disabled  FilterICVariant=InternalICsFilter  IntegratorICVariant=InternalICs  ExternalResetVariant=Disabled  TRSumVariant=Passthrough  SumFdbkVariant=Disabled  SumVariant=Sum_PID  TsampFilterVariant=InternalTs  TsampNgainVariant=Passthrough  TsampIntegralVariant=Disabled_SignalSpec  ExternalSaturationOutDataTypeStr=Inherit: Same as second input
      settings: LibrarySourceBlock=simulink/Discrete/Discrete PID Controller
  cfblk4 : DiscreteIntegrator  ICPrevOutput=DiscIntNeverNeededParam  ICPrevScaledInput=DiscIntNeverNeededParam
  cfblk5 : DiscreteIntegrator  ICPrevOutput=DiscIntNeverNeededParam  ICPrevScaledInput=DiscIntNeverNeededParam
  cfblk6 : DiscreteIntegrator  ICPrevOutput=DiscIntNeverNeededParam  ICPrevScaledInput=DiscIntNeverNeededParam
  cfblk7 : Sin  TimeSource=Use external signal  SampleTime=0
  cfblk8 : Reshape
  cfblk9 : Sum  Inputs=+
  cfblk2 : Outport
  wires:
  cfblk17/1 -> cfblk9/1
  cfblk1/1 -> cfblk6/1
  cfblk14/1(cfblk2) -> cfblk5/1
  cfblk9/1 -> cfblk2/1
  cfblk12/1(cfblk2) -> cfblk8/1
  cfblk6/1 -> cfblk12/3(cfblk11)
  cfblk3/1 -> cfblk10/1, cfblk14/2(cfblk7)
  cfblk13/1(cfblk2) -> cfblk15/1(cfblk1)
  cfblk5/1 -> cfblk15/2(cfblk11)
  cfblk16/2(cfblk8) -> cfblk7/1
  cfblk12/2(cfblk12) -> cfblk10/2
  cfblk7/1 -> cfblk3/1
  cfblk12/3(cfblk13) -> cfblk13/1(cfblk1)
  cfblk11/1 -> cfblk15/3(cfblk12)
  cfblk12/4(cfblk14) -> cfblk13/2(cfblk10)
  cfblk10/1 -> cfblk14/1(cfblk1)
  cfblk12/5(cfblk15) -> cfblk4/1
  cfblk4/1 -> cfblk16/1(cfblk1), cfblk14/3(cfblk8)
  cfblk16/3(cfblk9) -> cfblk15/4(cfblk13)
  cfblk8/1 -> cfblk16/2(cfblk6)
  cfblk13/2(cfblk11) -> cfblk16/3(cfblk7)
  cfblk16/1(cfblk2) -> cfblk18/1
  cfblk18/1 -> cfblk12/1(cfblk1)
  cfblk15/1(cfblk2) -> cfblk19/1
  cfblk19/1 -> cfblk12/2(cfblk10)

== system sampleModel653/cfblk129 ==
  cfblk1 : Inport
  cfblk13 : Inport  Port=2
  cfblk10 : Subsystem
  cfblk11 : Subsystem
  cfblk12 : Subsystem
  cfblk{14..20} (7 alike) : Delay  SampleTime=1
  cfblk3 : simulink/Discrete/Transfer Fcn First Order  PoleZ=0.95  ICPrevOutput=0.0  DoSatur=off
  cfblk4 : slpidlib/PID Controller  Controller=PID  Form=Parallel  TimeDomain=Discrete-time  UseExternalTs=off  SampleTime=1  IntegratorMethod=Forward Euler  FilterMethod=Forward Euler  ControllerParametersSource=internal  P=1  I=1  UseKiTs=off  D=0  N=100  UseFilter=on  TunerSelectOption=Transfer Function Based (PID Tuner App)  InitialConditionSource=internal  InitialConditionForIntegrator=0  InitialConditionForFilter=0  DifferentiatorICPrevScaledInput=0  ExternalReset=none  TrackingMode=off  Kt=1  LimitOutput=off  SatLimitsSource=internal  UpperSaturationLimit=inf  LowerSaturationLimit=-inf  LinearizeAsGain=off  AntiWindupMode=none  Kb=1  LimitIntegrator=off  UpperIntegratorSaturationLimit=inf  LowerIntegratorSaturationLimit=-inf  POutMin=[]  POutMax=[]  IOutMin=[]  IOutMax=[]  DOutMin=[]  DOutMax=[]  NOutMin=[]  NOutMax=[]  SumOutMin=[]  SumOutMax=[]  SaturationOutMin=[]  SaturationOutMax=[]  PParamMin=[]  PParamMax=[]  IParamMin=[]  IParamMax=[]  DParamMin=[]  DParamMax=[]  NParamMin=[]  NParamMax=[]  KbParamMin=[]  KbParamMax=[]  KtParamMin=[]  KtParamMax=[]  KbOutMin=[]  KbOutMax=[]  KtOutMin=[]  KtOutMax=[]  IntegratorOutMin=[]  IntegratorOutMax=[]  FilterOutMin=[]  FilterOutMax=[]  SumI1OutMin=[]  SumI1OutMax=[]  SumI2OutMin=[]  SumI2OutMax=[]  SumI3OutMin=[]  SumI3OutMax=[]  SumI4OutMin=[]  SumI4OutMax=[]  SumDOutMin=[]  SumDOutMax=[]  DifferentiatorOutMin=[]  DifferentiatorOutMax=[]  FilterDiffOutCoefMin=[]  FilterDiffOutCoefMax=[]  ReciprocalOutMin=[]  ReciprocalOutMax=[]  SumDenOutMin=[]  SumDenOutMax=[]  SumNumOutMin=[]  SumNumOutMax=[]  DivideOutMin=[]  DivideOutMax=[]  UdiffTsProdOutMin=[]  UdiffTsProdOutMax=[]  NTsProdOutMin=[]  NTsProdOutMax=[]  UintegralTsProdOutMin=[]  UintegralTsProdOutMax=[]  UngainTsProdOutMin=[]  UngainTsProdOutMax=[]  ClampingZeroOutDataTypeStr=Inherit: Inherit via back propagation  ClampingZeroOutMin=[]  ClampingZeroOutMax=[]  FilterDenConstantOutDataTypeStr=Inherit: Inherit via back propagation  FilterDenConstantOutMin=[]  FilterDenConstantOutMax=[]  PCopyOutDataTypeStr=Inherit: Inherit via back propagation  PCopyOutMin=[]  PCopyOutMax=[]  NCopyOutDataTypeStr=Inherit: Inherit via back propagation  NCopyOutMin=[]  NCopyOutMax=[]  IntegratorContinuousStateAttributes=''  IntegratorStateMustResolveToSignalObject=off  IntegratorRTWStateStorageClass=Auto  FilterContinuousStateAttributes=''  FilterStateMustResolveToSignalObject=off  FilterRTWStateStorageClass=Auto  ParallelPVariant=InternalParameters  IdealPVariant=Disabled  IVariant=InternalParameters  DVariant=InternalParameters  IntegratorVariant=Discrete  SatVariant=Disabled  AWVariant=Passthrough  PCopyVariant=Disabled  TRVariant=Disabled  FdbkBlocksVariant=Forward  IdealPFdbkVariant=Disabled  SatFdbkVariant=Disabled  DerivativeFilterVariant=ForwardEulerFilter  NVariant=InternalParameters  NCopyVariant=Disabled  FilterICVariant=InternalICsFilter  IntegratorICVariant=InternalICs  ExternalResetVariant=Disabled  TRSumVariant=Passthrough  SumFdbkVariant=Disabled  SumVariant=Sum_PID  TsampFilterVariant=InternalTs  TsampNgainVariant=Passthrough  TsampIntegralVariant=Disabled_SignalSpec  ExternalSaturationOutDataTypeStr=Inherit: Same as second input
      settings: LibrarySourceBlock=simulink/Discrete/Discrete PID Controller
  cfblk5 : DiscreteIntegrator  ICPrevOutput=DiscIntNeverNeededParam  ICPrevScaledInput=DiscIntNeverNeededParam
  cfblk6 : slpidlib/PID Controller  Controller=PID  Form=Parallel  TimeDomain=Discrete-time  UseExternalTs=off  SampleTime=1  IntegratorMethod=Forward Euler  FilterMethod=Forward Euler  ControllerParametersSource=internal  P=1  I=1  UseKiTs=off  D=0  N=100  UseFilter=on  TunerSelectOption=Transfer Function Based (PID Tuner App)  InitialConditionSource=internal  InitialConditionForIntegrator=0  InitialConditionForFilter=0  DifferentiatorICPrevScaledInput=0  ExternalReset=none  TrackingMode=off  Kt=1  LimitOutput=off  SatLimitsSource=internal  UpperSaturationLimit=inf  LowerSaturationLimit=-inf  LinearizeAsGain=off  AntiWindupMode=none  Kb=1  LimitIntegrator=off  UpperIntegratorSaturationLimit=inf  LowerIntegratorSaturationLimit=-inf  POutMin=[]  POutMax=[]  IOutMin=[]  IOutMax=[]  DOutMin=[]  DOutMax=[]  NOutMin=[]  NOutMax=[]  SumOutMin=[]  SumOutMax=[]  SaturationOutMin=[]  SaturationOutMax=[]  PParamMin=[]  PParamMax=[]  IParamMin=[]  IParamMax=[]  DParamMin=[]  DParamMax=[]  NParamMin=[]  NParamMax=[]  KbParamMin=[]  KbParamMax=[]  KtParamMin=[]  KtParamMax=[]  KbOutMin=[]  KbOutMax=[]  KtOutMin=[]  KtOutMax=[]  IntegratorOutMin=[]  IntegratorOutMax=[]  FilterOutMin=[]  FilterOutMax=[]  SumI1OutMin=[]  SumI1OutMax=[]  SumI2OutMin=[]  SumI2OutMax=[]  SumI3OutMin=[]  SumI3OutMax=[]  SumI4OutMin=[]  SumI4OutMax=[]  SumDOutMin=[]  SumDOutMax=[]  DifferentiatorOutMin=[]  DifferentiatorOutMax=[]  FilterDiffOutCoefMin=[]  FilterDiffOutCoefMax=[]  ReciprocalOutMin=[]  ReciprocalOutMax=[]  SumDenOutMin=[]  SumDenOutMax=[]  SumNumOutMin=[]  SumNumOutMax=[]  DivideOutMin=[]  DivideOutMax=[]  UdiffTsProdOutMin=[]  UdiffTsProdOutMax=[]  NTsProdOutMin=[]  NTsProdOutMax=[]  UintegralTsProdOutMin=[]  UintegralTsProdOutMax=[]  UngainTsProdOutMin=[]  UngainTsProdOutMax=[]  ClampingZeroOutDataTypeStr=Inherit: Inherit via back propagation  ClampingZeroOutMin=[]  ClampingZeroOutMax=[]  FilterDenConstantOutDataTypeStr=Inherit: Inherit via back propagation  FilterDenConstantOutMin=[]  FilterDenConstantOutMax=[]  PCopyOutDataTypeStr=Inherit: Inherit via back propagation  PCopyOutMin=[]  PCopyOutMax=[]  NCopyOutDataTypeStr=Inherit: Inherit via back propagation  NCopyOutMin=[]  NCopyOutMax=[]  IntegratorContinuousStateAttributes=''  IntegratorStateMustResolveToSignalObject=off  IntegratorRTWStateStorageClass=Auto  FilterContinuousStateAttributes=''  FilterStateMustResolveToSignalObject=off  FilterRTWStateStorageClass=Auto  ParallelPVariant=InternalParameters  IdealPVariant=Disabled  IVariant=InternalParameters  DVariant=InternalParameters  IntegratorVariant=Discrete  SatVariant=Disabled  AWVariant=Passthrough  PCopyVariant=Disabled  TRVariant=Disabled  FdbkBlocksVariant=Forward  IdealPFdbkVariant=Disabled  SatFdbkVariant=Disabled  DerivativeFilterVariant=ForwardEulerFilter  NVariant=InternalParameters  NCopyVariant=Disabled  FilterICVariant=InternalICsFilter  IntegratorICVariant=InternalICs  ExternalResetVariant=Disabled  TRSumVariant=Passthrough  SumFdbkVariant=Disabled  SumVariant=Sum_PID  TsampFilterVariant=InternalTs  TsampNgainVariant=Passthrough  TsampIntegralVariant=Disabled_SignalSpec  ExternalSaturationOutDataTypeStr=Inherit: Same as second input
      settings: LibrarySourceBlock=simulink/Discrete/Discrete PID Controller
  cfblk7 : Assignment  DiagnosticForDimensions=Warning  IndexOptions=Index vector (dialog)  Indices=1  OutputSizes=1
  cfblk8 : DotProduct  OutDataTypeStr=Inherit: Inherit via internal rule
  cfblk9 : Subsystem
  cfblk2 : Outport
  wires:
  cfblk11/1(cfblk2) -> cfblk2/1
  cfblk3/1 -> cfblk17/1, cfblk18/1
  cfblk6/1 -> cfblk3/1, cfblk19/1
  cfblk8/1 -> cfblk12/3(cfblk10)
  cfblk7/1 -> cfblk11/2(cfblk10), cfblk14/1
  cfblk11/2(cfblk12) -> cfblk9/1(cfblk1)
  cfblk1/1 -> cfblk8/2
  cfblk11/3(cfblk13) -> cfblk9/2(cfblk9)
  cfblk10/1(cfblk2) -> cfblk6/1
  cfblk12/1(cfblk2) -> cfblk7/2
  cfblk13/1 -> cfblk9/3(cfblk10), cfblk11/3(cfblk11)
  cfblk11/4(cfblk14) -> cfblk5/1, cfblk4/1
  cfblk9/2(cfblk11) -> cfblk10/2(cfblk8), cfblk16/1
  cfblk5/1 -> cfblk10/1(cfblk1)
  cfblk14/1 -> cfblk8/1
  cfblk9/1(cfblk2) -> cfblk15/1
  cfblk15/1 -> cfblk12/2(cfblk9)
  cfblk16/1 -> cfblk11/1(cfblk1)
  cfblk17/1 -> cfblk12/1(cfblk1)
  cfblk18/1 -> cfblk10/4(cfblk10)
  cfblk19/1 -> cfblk10/3(cfblk9)
  cfblk4/1 -> cfblk20/1
  cfblk20/1 -> cfblk7/1

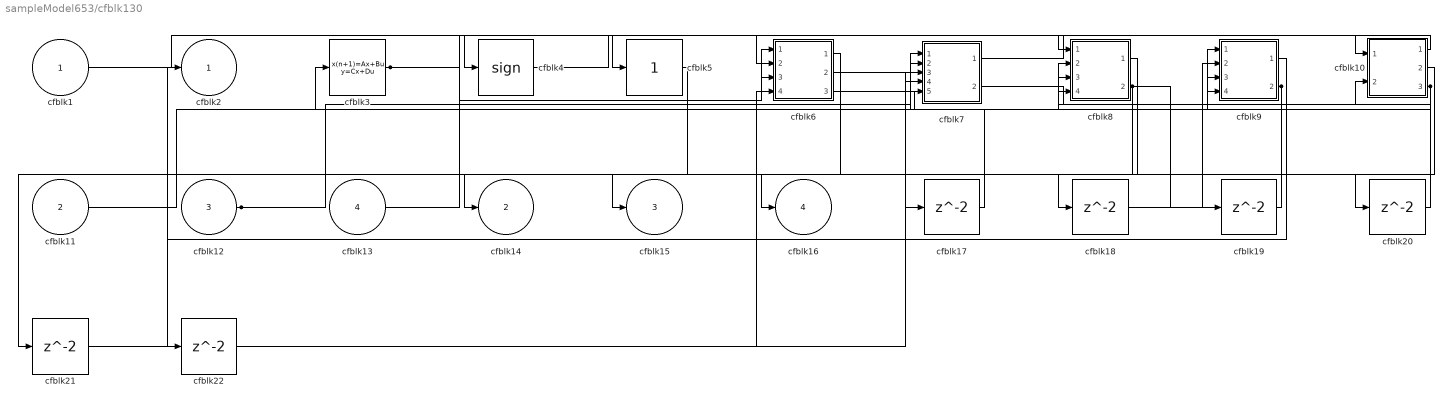
== system sampleModel653/cfblk130 ==
  cfblk1 : Inport
  cfblk11 : Inport  Port=2
  cfblk12 : Inport  Port=3
  cfblk13 : Inport  Port=4
  cfblk10 : Subsystem
  cfblk{17..22} (6 alike) : Delay  SampleTime=1
  cfblk3 : DiscreteStateSpace
  cfblk4 : Signum
  cfblk5 : simulink/Math Operations/Slider Gain  gain=1  low=0  high=2
  cfblk6 : Subsystem
  cfblk7 : Subsystem
  cfblk8 : Subsystem
  cfblk9 : Subsystem
  cfblk2 : Outport
  cfblk14 : Outport  Port=2
  cfblk15 : Outport  Port=3
  cfblk16 : Outport  Port=4
  wires:
  cfblk7/1(cfblk2) -> cfblk10/1(cfblk1)
  cfblk12/1 -> cfblk7/1(cfblk1), cfblk8/3(cfblk9), cfblk9/4(cfblk14)
  cfblk1/1 -> cfblk5/1
  cfblk5/1 -> cfblk14/1
  cfblk9/1(cfblk2) -> cfblk2/1
  cfblk11/1 -> cfblk9/1(cfblk1)
  cfblk7/2(cfblk17) -> cfblk10/2(cfblk10)
  cfblk6/1(cfblk2) -> cfblk16/1
  cfblk4/1 -> cfblk8/1(cfblk1)
  cfblk13/1 -> cfblk6/1(cfblk1)
  cfblk10/1(cfblk2) -> cfblk4/1
  cfblk9/2(cfblk15) -> cfblk7/2(cfblk13), cfblk22/1
  cfblk8/2(cfblk11) -> cfblk15/1, cfblk19/1
  cfblk3/1 -> cfblk6/2(cfblk6), cfblk6/3(cfblk7)
  cfblk6/3(cfblk10) -> cfblk9/3(cfblk13)
  cfblk10/3(cfblk12) -> cfblk8/2(cfblk8), cfblk8/4(cfblk10), cfblk21/1
  cfblk6/2(cfblk9) -> cfblk17/1
  cfblk17/1 -> cfblk3/1
  cfblk8/1(cfblk2) -> cfblk18/1
  cfblk18/1 -> cfblk9/2(cfblk12)
  cfblk19/1 -> cfblk7/4(cfblk15)
  cfblk10/2(cfblk11) -> cfblk20/1
  cfblk20/1 -> cfblk7/3(cfblk14)
  cfblk21/1 -> cfblk7/5(cfblk16)
  cfblk22/1 -> cfblk6/4(cfblk8)

== system sampleModel653/cfblk131 ==
  cfblk1 : Inport
  cfblk14 : Inport  Port=2
  cfblk15 : Inport  Port=3
  cfblk10 : Gain  Gain=[155015884.290844]
  cfblk11 : Polyval  Coefs=[ +2.081618890e-019, -1.441693666e-014, +4.719686976e-010, -8.536869453e-006, +1.621573104e-001, -8.087801117e+001 ]
  cfblk12 : Subsystem
  cfblk13 : Subsystem
  cfblk16 : Delay  SampleTime=1
  cfblk17 : Delay  SampleTime=1
  cfblk18 : Delay  SampleTime=1
  cfblk3 : simulink/Discrete/Transfer Fcn Real Zero  ZeroZ=0.75  ICPrevInput=0.0  DoSatur=off
  cfblk4 : simulink/Discrete/Transfer Fcn Real Zero  ZeroZ=0.75  ICPrevInput=0.0  DoSatur=off
  cfblk5 : simulink/Discrete/Transfer Fcn First Order  PoleZ=0.95  ICPrevOutput=0.0  DoSatur=off
  cfblk6 : simulink/Discrete/Tapped Delay  vinit=0.0  samptime=-1  NumDelays=1  DelayOrder=Oldest  includeCurrent=off
  cfblk7 : simulink/Math Operations/MinMax Running Resettable  Function=min  vinit=0.0
  cfblk8 : Reshape
  cfblk9 : Sum  Inputs=+-
  cfblk2 : Outport
  wires:
  cfblk15/1 -> cfblk3/1
  cfblk11/1 -> cfblk10/1
  cfblk7/1 -> cfblk13/1(cfblk1)
  cfblk4/1 -> cfblk5/1
  cfblk9/1 -> cfblk12/1(cfblk1)
  cfblk13/1(cfblk2) -> cfblk9/1
  cfblk6/1 -> cfblk2/1
  cfblk3/1 -> cfblk4/1
  cfblk12/1(cfblk2) -> cfblk8/1
  cfblk14/1 -> cfblk6/1
  cfblk5/1 -> cfblk7/2
  cfblk12/3(cfblk16) -> cfblk11/1
  cfblk8/1 -> cfblk16/1
  cfblk16/1 -> cfblk12/2(cfblk14)
  cfblk12/2(cfblk15) -> cfblk17/1
  cfblk17/1 -> cfblk7/1
  cfblk10/1 -> cfblk18/1
  cfblk18/1 -> cfblk9/2

== system sampleModel653/cfblk132 ==
  cfblk1 : Inport
  cfblk10 : Subsystem
  cfblk11 : Subsystem
  cfblk12 : Subsystem
  cfblk15 : Delay  SampleTime=1
  cfblk16 : Delay  SampleTime=1
  cfblk17 : Delay  SampleTime=1
  cfblk3 : simulink/Discrete/Tapped Delay  vinit=0.0  samptime=-1  NumDelays=1  DelayOrder=Oldest  includeCurrent=off
  cfblk4 : Delay  DelayLengthSource=Input port  SampleTime=1
      settings: InputPortMap=u0,p1
  cfblk5 : DiscreteFir  SampleTime=1
  cfblk6 : Squeeze
  cfblk7 : Math  Operator=square
  cfblk8 : ComplexToRealImag
  cfblk9 : Constant  Value=[-325607633.525440]  SampleTime=1
  cfblk2 : Outport
  cfblk13 : Outport  Port=2
  cfblk14 : Outport  Port=3
  wires:
  cfblk6/1 -> cfblk5/1
  cfblk10/1(cfblk2) -> cfblk2/1
  cfblk8/1 -> cfblk3/1
  cfblk10/2(cfblk15) -> cfblk4/1
  cfblk12/1(cfblk2) -> cfblk6/1
  cfblk10/3(cfblk16) -> cfblk14/1, cfblk11/4(cfblk9), cfblk11/5(cfblk10)
  cfblk4/1 -> cfblk8/1
  cfblk1/1 -> cfblk10/1(cfblk1), cfblk10/4(cfblk14)
  cfblk9/1 -> cfblk7/1
  cfblk8/2 -> cfblk11/1(cfblk1)
  cfblk3/1 -> cfblk12/1(cfblk1)
  cfblk7/1 -> cfblk11/2(cfblk7)
  cfblk11/2(cfblk11) -> cfblk13/1, cfblk16/1
  cfblk5/1 -> cfblk11/3(cfblk8)
  cfblk11/1(cfblk2) -> cfblk15/1
  cfblk15/1 -> cfblk10/2(cfblk12)
  cfblk16/1 -> cfblk10/3(cfblk13)
  cfblk12/2(cfblk7) -> cfblk17/1
  cfblk17/1 -> cfblk4/2

== system sampleModel653/cfblk133 ==
  cfblk1 : Inport
  cfblk7 : Inport  Port=2
  cfblk8 : Inport  Port=3
  cfblk9 : Inport  Port=4
  cfblk11 : Subsystem  TreatAsAtomicUnit=on
  cfblk12 : Subsystem  TreatAsAtomicUnit=on
  cfblk13 : Delay  SampleTime=1
  cfblk3 : Constant  Value=[128029269.683548]  SampleTime=1
  cfblk4 : Subsystem
  cfblk5 : Subsystem
  cfblk6 : If  IfExpression=u1 >= 0  SampleTime=1
  cfblk2 : Outport
  cfblk10 : Outport  Port=2
  wires:
  cfblk7/1 -> cfblk6/1, cfblk12/3(cfblk15)
  cfblk9/1 -> cfblk10/1, cfblk4/1(cfblk1)
  cfblk4/1(cfblk2) -> cfblk11/1(cfblk1)
  cfblk11/1(cfblk2) -> cfblk2/1
  cfblk3/1 -> cfblk5/1(cfblk1)
  cfblk12/1(cfblk2) -> cfblk5/2(cfblk10)
  cfblk8/1 -> cfblk5/3(cfblk11)
  cfblk1/1 -> cfblk12/2(cfblk14)
  cfblk12/2(cfblk16) -> cfblk5/4(cfblk12), cfblk5/5(cfblk13)
  cfblk6/1 -> cfblk11/Action
  cfblk6/2 -> cfblk12/Action
  cfblk5/1(cfblk2) -> cfblk13/1
  cfblk13/1 -> cfblk12/1(cfblk1)

== system sampleModel653/cfblk134 ==
  cfblk1 : Inport
  cfblk9 : Inport  Port=2
  cfblk10 : Delay  SampleTime=1
  cfblk11 : Delay  SampleTime=1
  cfblk3 : slpidlib/PID Controller  Controller=PID  Form=Parallel  TimeDomain=Discrete-time  UseExternalTs=off  SampleTime=1  IntegratorMethod=Forward Euler  FilterMethod=Forward Euler  ControllerParametersSource=internal  P=1  I=1  UseKiTs=off  D=0  N=100  UseFilter=on  TunerSelectOption=Transfer Function Based (PID Tuner App)  InitialConditionSource=internal  InitialConditionForIntegrator=0  InitialConditionForFilter=0  DifferentiatorICPrevScaledInput=0  ExternalReset=none  TrackingMode=off  Kt=1  LimitOutput=off  SatLimitsSource=internal  UpperSaturationLimit=inf  LowerSaturationLimit=-inf  LinearizeAsGain=off  AntiWindupMode=none  Kb=1  LimitIntegrator=off  UpperIntegratorSaturationLimit=inf  LowerIntegratorSaturationLimit=-inf  POutMin=[]  POutMax=[]  IOutMin=[]  IOutMax=[]  DOutMin=[]  DOutMax=[]  NOutMin=[]  NOutMax=[]  SumOutMin=[]  SumOutMax=[]  SaturationOutMin=[]  SaturationOutMax=[]  PParamMin=[]  PParamMax=[]  IParamMin=[]  IParamMax=[]  DParamMin=[]  DParamMax=[]  NParamMin=[]  NParamMax=[]  KbParamMin=[]  KbParamMax=[]  KtParamMin=[]  KtParamMax=[]  KbOutMin=[]  KbOutMax=[]  KtOutMin=[]  KtOutMax=[]  IntegratorOutMin=[]  IntegratorOutMax=[]  FilterOutMin=[]  FilterOutMax=[]  SumI1OutMin=[]  SumI1OutMax=[]  SumI2OutMin=[]  SumI2OutMax=[]  SumI3OutMin=[]  SumI3OutMax=[]  SumI4OutMin=[]  SumI4OutMax=[]  SumDOutMin=[]  SumDOutMax=[]  DifferentiatorOutMin=[]  DifferentiatorOutMax=[]  FilterDiffOutCoefMin=[]  FilterDiffOutCoefMax=[]  ReciprocalOutMin=[]  ReciprocalOutMax=[]  SumDenOutMin=[]  SumDenOutMax=[]  SumNumOutMin=[]  SumNumOutMax=[]  DivideOutMin=[]  DivideOutMax=[]  UdiffTsProdOutMin=[]  UdiffTsProdOutMax=[]  NTsProdOutMin=[]  NTsProdOutMax=[]  UintegralTsProdOutMin=[]  UintegralTsProdOutMax=[]  UngainTsProdOutMin=[]  UngainTsProdOutMax=[]  ClampingZeroOutDataTypeStr=Inherit: Inherit via back propagation  ClampingZeroOutMin=[]  ClampingZeroOutMax=[]  FilterDenConstantOutDataTypeStr=Inherit: Inherit via back propagation  FilterDenConstantOutMin=[]  FilterDenConstantOutMax=[]  PCopyOutDataTypeStr=Inherit: Inherit via back propagation  PCopyOutMin=[]  PCopyOutMax=[]  NCopyOutDataTypeStr=Inherit: Inherit via back propagation  NCopyOutMin=[]  NCopyOutMax=[]  IntegratorContinuousStateAttributes=''  IntegratorStateMustResolveToSignalObject=off  IntegratorRTWStateStorageClass=Auto  FilterContinuousStateAttributes=''  FilterStateMustResolveToSignalObject=off  FilterRTWStateStorageClass=Auto  ParallelPVariant=InternalParameters  IdealPVariant=Disabled  IVariant=InternalParameters  DVariant=InternalParameters  IntegratorVariant=Discrete  SatVariant=Disabled  AWVariant=Passthrough  PCopyVariant=Disabled  TRVariant=Disabled  FdbkBlocksVariant=Forward  IdealPFdbkVariant=Disabled  SatFdbkVariant=Disabled  DerivativeFilterVariant=ForwardEulerFilter  NVariant=InternalParameters  NCopyVariant=Disabled  FilterICVariant=InternalICsFilter  IntegratorICVariant=InternalICs  ExternalResetVariant=Disabled  TRSumVariant=Passthrough  SumFdbkVariant=Disabled  SumVariant=Sum_PID  TsampFilterVariant=InternalTs  TsampNgainVariant=Passthrough  TsampIntegralVariant=Disabled_SignalSpec  ExternalSaturationOutDataTypeStr=Inherit: Same as second input
      settings: LibrarySourceBlock=simulink/Discrete/Discrete PID Controller
  cfblk4 : simulink/Math Operations/MinMax Running Resettable  Function=min  vinit=0.0
  cfblk5 : UnaryMinus
  cfblk6 : Sum  Inputs=+-
  cfblk7 : Subsystem
  cfblk8 : Subsystem
  cfblk2 : Outport
  wires:
  cfblk7/1(cfblk2) -> cfblk2/1
  cfblk6/1 -> cfblk3/1, cfblk8/2(cfblk12)
  cfblk8/1(cfblk2) -> cfblk4/1
  cfblk9/1 -> cfblk8/1(cfblk1)
  cfblk1/1 -> cfblk5/1, cfblk7/5(cfblk12)
  cfblk5/1 -> cfblk7/1(cfblk1), cfblk6/2, cfblk7/3(cfblk10)
  cfblk3/1 -> cfblk4/2, cfblk11/1
  cfblk7/2(cfblk13) -> cfblk6/1
  cfblk4/1 -> cfblk10/1
  cfblk10/1 -> cfblk7/2(cfblk9)
  cfblk11/1 -> cfblk7/4(cfblk11)
